simulink model "test_L_detector"  (Simulink 7.6)
settings: Solver=FixedStepDiscrete  StartTime=0.0  StopTime=0  RelTol=1e-3
values from neighbouring files (symbols this model uses):
  Forward_Camera_Dimensions = [640 480]    [VisionConstants.m]
  Iter_Segment_Thresh = 60    [VisionConstants.m]
  Scale_Forward_B = 1    [VisionConstants.m]
  Scale_Forward_G = 1    [VisionConstants.m]
  Scale_Forward_H = .8    (= 0.8)    [VisionConstants.m]
  Scale_Forward_R = 1    [VisionConstants.m]
  Scale_Forward_S = 1    [VisionConstants.m]
  Scale_Forward_V = 2    [VisionConstants.m]
undefined symbols (not defined in the file or in its folder): black_al, black_au, black_bl, black_bu, blue_al, blue_au, blue_bl, blue_bu, Forward_Fov, gray, green_al, green_au, green_bl, green_bu, orange_al, orange_au, orange_bl, orange_bu, Rec, red_al, red_au, red_bl, red_bu, SDTV, white_al, white_au, white_bl, white_bu, yellow_al, yellow_au, yellow_bl, yellow_bu
libraries: vipconversions x4, vipgeotforms x3, viptextngfix x2, vipsnks x2, viptransforms x2, vipanalysis x1, vipsrcs x1
(part 2 of 2)

== matlab function Blob_Analysis/make_color_range ==
  data: a_range output double; b_range output double; white_al input double; white_au input double; white_bl input double; white_bu input double; black_al input double; black_au input double; black_bl input double; black_bu input double; blue_al input double; blue_au input double; blue_bl input double; blue_bu input double; red_al input double; red_au input double; red_bl input double; red_bu input double; orange_al input double; orange_au input double; orange_bl input double; orange_bu input double; yellow_al input double; yellow_au input double; yellow_bl input double; yellow_bu input double; green_al input double; green_au input double; green_bl input double; green_bu input double
function [a_range, b_range] = make_color_range(white_al, white_au, white_bl, white_bu, black_al, black_au, black_bl, black_bu, blue_al, blue_au, blue_bl, blue_bu, red_al, red_au, red_bl, red_bu, orange_al, orange_au, orange_bl, orange_bu, yellow_al, yellow_au, yellow_bl, yellow_bu, green_al, green_au, green_bl, green_bu)

% This function forms two compact matrices which pass all color range
%   information to other functions in the model


% Initialize
a_range = zeros(2, 7);
b_range = zeros(2, 7);


% Assign values to color range matrices
a_range(1, 1) = white_al;
a_range(2, 1) = white_au;
b_range(1, 1) = white_bl;
b_range(2, 1) = white_bu;

a_range(1, 2) = black_al;
a_range(2, 2) = black_au;
b_range(1, 2) = black_bl;
b_range(2, 2) = black_bu;

a_range(1, 3) = blue_al;
a_range(2, 3) = blue_au;
b_range(1, 3) = blue_bl;
b_range(2, 3) = blue_bu;

a_range(1, 4) = red_al;
a_range(2, 4) = red_au;
b_range(1, 4) = red_bl;
b_range(2, 4) = red_bu;

a_range(1, 5) = orange_al;
a_range(2, 5) = orange_au;
b_range(1, 5) = orange_bl;
b_range(2, 5) = orange_bu;

a_range(1, 6) = yellow_al;
a_range(2, 6) = yellow_au;
b_range(1, 6) = yellow_bl;
b_range(2, 6) = yellow_bu;

a_range(1, 7) = green_al;
a_range(2, 7) = green_au;
b_range(1, 7) = green_bl;
b_range(2, 7) = green_bu;


return
